simulink model "ModeloFogueteSimulink"  (R2019a)
settings: Solver=VariableStepAuto  StartTime=0.0  StopTime=160  RelTol=1e-3
undefined symbols (not defined in the file): A, B, C
settings Model: Creator=Cliente  LastModifiedBy=Cliente

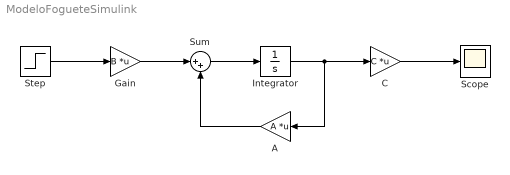
== system ModeloFogueteSimulink ==
  A : Gain  Gain=A  Multiplication=Matrix(K*u) (u vector)
  C : Gain  Gain=C  Multiplication=Matrix(K*u) (u vector)
  Gain : Gain  Gain=B  Multiplication=Matrix(K*u)
  Integrator : Integrator  InitialCondition=[1.58;0]
  Scope : Scope
  Step : Step  Time=0.05  Before=-365  After=10  SampleTime=1
  Sum : Sum  Inputs=|++
  wires:
  C/1 -> Scope/1
  Integrator/1 -> A/1, C/1
  A/1 -> Sum/2
  Sum/1 -> Integrator/1
  Gain/1 -> Sum/1
  Step/1 -> Gain/1
